simulink model "LaserLocker"  (R2017a)
settings: Solver=VariableStepAuto  StartTime=0.0  StopTime=10.0  RelTol=1e-3
libraries: arduinolib x3, powerlib_meascontrol x1
settings Model: Creator=Stuart Smyth  LastModifiedBy=Stuart Smyth

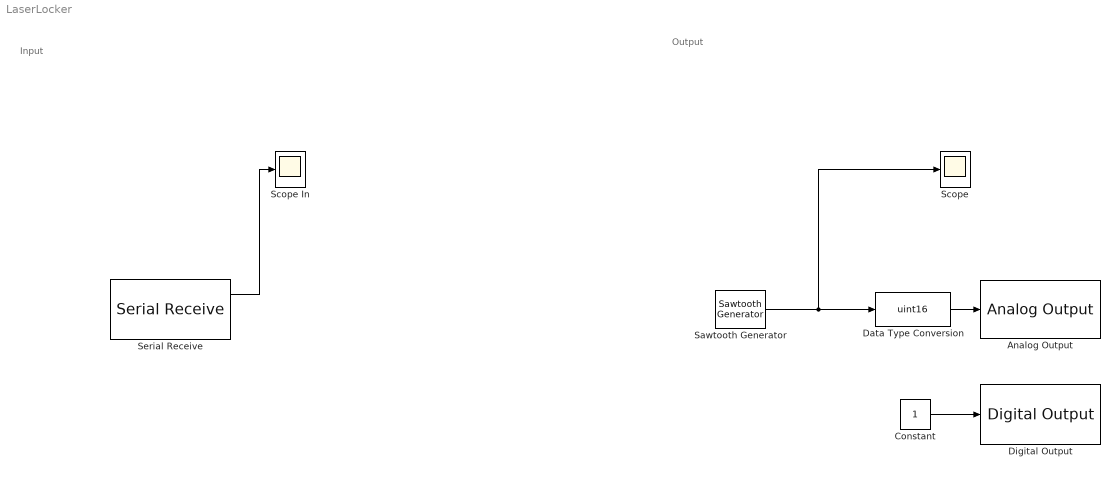
== system LaserLocker ==
  note: Input
  note: Output
  Analog Output : arduinolib/Analog Output  DACpin=DAC0  blockPlatform=arduino
      settings: SourceProductName=Simulink Support Package for Arduino Hardware  SourceProductBaseCode=ARDUINO
  Constant : Constant
  Data Type Conversion : DataTypeConversion  OutDataTypeStr=uint16
  Digital Output : arduinolib/Digital Output  pinNumber=9  blockPlatform=arduino
  Sawtooth Generator : powerlib_meascontrol/Pulse & Signal Generators/Sawtooth Generator  Freq=10  Phase=180  Ts=0
      settings: SourceProductName=Simscape Power Systems
  Scope : Scope
  Scope In : Scope
  Serial Receive : arduinolib/Serial Receive  isARMArch=off  portNumber=0  DataType=uint8  Datalength=1  SampleTime=0.1  showOutStatus=on  blockPlatform=arduino
      settings: SourceProductName=Simulink Support Package for Arduino Hardware  SourceProductBaseCode=ARDUINO
  wires:
  Data Type Conversion/1 -> Analog Output/1
  Sawtooth Generator/1 -> Data Type Conversion/1, Scope/1
  Serial Receive/1 -> Scope In/1
  Constant/1 -> Digital Output/1
